simulink model "vertMotorSimMath"  (R2024b)
settings: Solver=FixedStepDiscrete  StartTime=0.0  StopTime=inf  FixedStep=0.002  RelTol=1e-3  EnableMultiTasking=on
undefined symbols (not defined in the file or in its folder): prop, rad, s
libraries: aerolibconvert2 x1
settings Model: ExtModeTrigDuration=10000  Creator=jellu  LastModifiedBy=jellu
settings SolverCC: AlgebraicLoopSolver=TrustRegion  PositivePriorityOrder=on
settings DataIOCC: ReturnWorkspaceOutputs=off
settings OptimizationCC: LifeSpan=inf
settings DebuggingCC: UnconnectedInputMsg=warning  UnconnectedOutputMsg=warning  UnconnectedLineMsg=warning  ArithmeticOperatorsInVariantConditions=warning
settings ModelReferenceCC: EnableRefExpFcnMdlSchedulingChecks=on
settings SFSimCC: SimUseLocalCustomCode=off  CustomCodeUndefinedFunction=UseInterfaceOnly
settings RTWCC: Description=QUARC Win64 Target  SystemTargetFile=quarc_win64.tlc  TemplateMakefile=quarc_default_tmf  RTWUseLocalCustomCode=off  GPUComputeCapability=3.5
settings CodeAppCC: StateflowObjectComments=on
settings STFCustomTargetCC: TargetPreCompLibLocation=C:\PROGRA~3\QUARC\lib\2016a\win64\release  TargetLangStandard=C99 (ISO)  ConcurrentExecutionCompliant=on  GRTInterface=on  SystemTargetFile=quarc_win64.tlc
settings GRTTargetCC: TargetPreCompLibLocation=C:\PROGRA~3\QUARC\lib\2016a\win64\release  ParMdlRefBuildCompliant=off  CompOptLevelCompliant=off  CombineOutputUpdateFcns=off  MatFileLogging=off  CPPClassGenCompliant=off  GRTInterface=on  UseToolchainInfoCompliant=off  ExtMode=on  ExtModeMexFile=quarc_comm
settings ConfigComp: CovMetricSettings=dswe

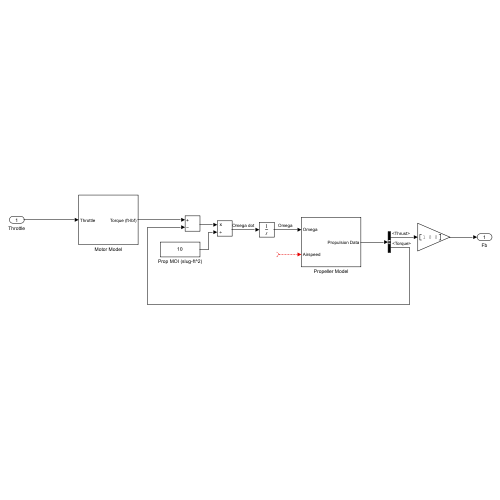
[thumbnail: Simulink's stored preview of the top-level diagram]
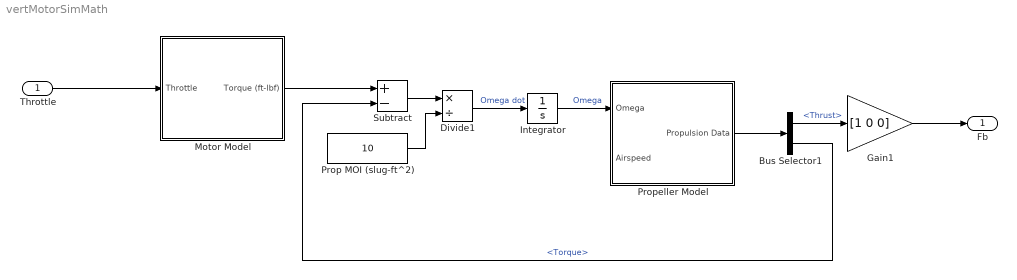
== system vertMotorSimMath ==
  Throttle : Inport
  Bus Selector1 : BusSelector  OutputSignals=Thrust,Torque
  Divide1 : Product  Inputs=*/
  Gain1 : Gain  Gain=[1 0 0]
  Integrator : Integrator  InitialCondition=200
  Motor Model : Subsystem
  Prop MOI (slug-ft^2) : Constant  Value=10
  Propeller Model : Subsystem
  Subtract : Sum  Inputs=+-
  Fb : Outport
  wires:
  Divide1/1 -> Integrator/1  "Omega dot"
  Integrator/1 -> Propeller Model/1(Omega)  "Omega"
  Gain1/1 -> Fb/1
  Motor Model/1(Torque (ft-lbf)) -> Subtract/1
  ? -> Propeller Model/2(Airspeed)
  Bus Selector1/2 -> Subtract/2  "<Torque>"
  Bus Selector1/1 -> Gain1/1  "<Thrust>"
  Prop MOI (slug-ft^2)/1 -> Divide1/2
  Subtract/1 -> Divide1/1
  Propeller Model/1(Propulsion Data) -> Bus Selector1/1
  Throttle/1 -> Motor Model/1(Throttle)

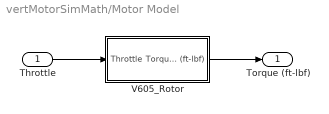
== system vertMotorSimMath/Motor Model ==
  Throttle : Inport
  V605_Rotor : Subsystem
  Torque (ft-lbf) : Outport
  wires:
  V605_Rotor/1(Torque (ft-lbf)) -> Torque (ft-lbf)/1
  Throttle/1 -> V605_Rotor/1(Throttle)

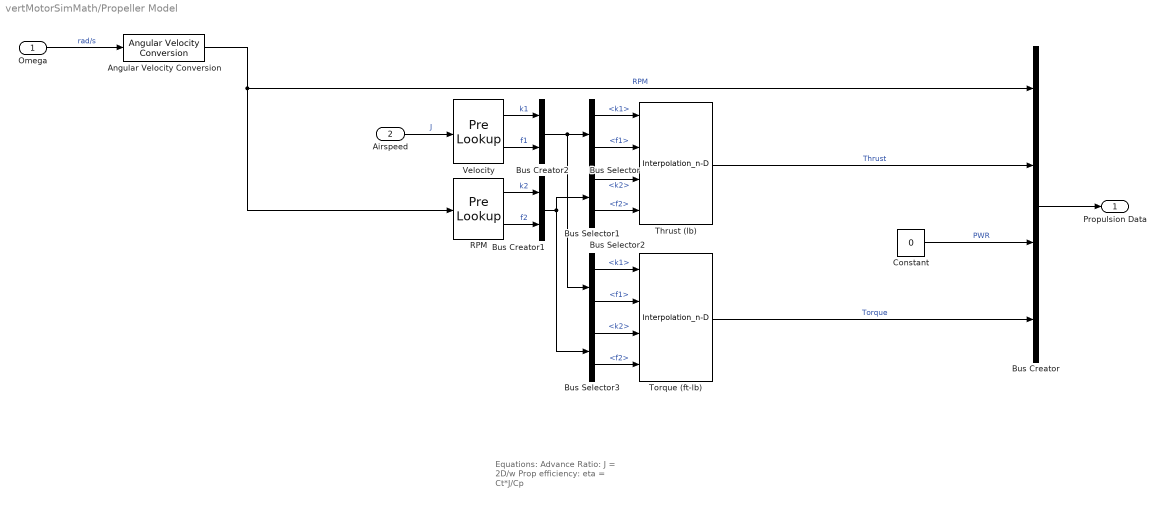
== system vertMotorSimMath/Propeller Model ==
  note: Equations:
      |
      | Advance Ratio: J = 2D/w
      | Prop efficiency: eta = Ct*J/Cp
  Omega : Inport
  Airspeed : Inport  Port=2
  Angular Velocity Conversion : aerolibconvert2/Angular Velocity Conversion  IU=rad/s  OU=rpm
  Bus Creator : BusCreator  Inputs=4
  Bus Creator1 : BusCreator  Inputs=2
  Bus Creator2 : BusCreator  Inputs=2
  Bus Selector : BusSelector  OutputSignals=k1,f1
  Bus Selector1 : BusSelector  OutputSignals=k2,f2
  Bus Selector2 : BusSelector  OutputSignals=k1,f1
  Bus Selector3 : BusSelector  OutputSignals=k2,f2
  Constant : Constant  Value=0
  RPM : PreLookup  BreakpointsData=prop.RPM  ExtrapMethod=Linear
  Thrust (lb) : Interpolation_n-D  Table=prop.Thrust  InternalRulePriority=Speed
  Torque (ft-lb) : Interpolation_n-D  Table=prop.Torque  ExtrapMethod=Clip  InternalRulePriority=Speed
  Velocity : PreLookup  BreakpointsData=prop.vel
  Propulsion Data : Outport
  wires:
  Constant/1 -> Bus Creator/3  "PWR"
  Torque (ft-lb)/1 -> Bus Creator/4  "Torque"
  Angular Velocity Conversion/1 -> RPM/1, Bus Creator/1  "RPM"
  Bus Creator/1 -> Propulsion Data/1
  Omega/1 -> Angular Velocity Conversion/1  "rad/s"
  Airspeed/1 -> Velocity/1  "J"
  Velocity/2 -> Bus Creator2/2  "f1"
  Bus Creator2/1 -> Bus Selector/1, Bus Selector2/1
  Bus Creator1/1 -> Bus Selector1/1, Bus Selector3/1
  Velocity/1 -> Bus Creator2/1  "k1"
  Bus Selector2/2 -> Torque (ft-lb)/2  "<f1>"
  RPM/1 -> Bus Creator1/1  "k2"
  Bus Selector2/1 -> Torque (ft-lb)/1  "<k1>"
  RPM/2 -> Bus Creator1/2  "f2"
  Thrust (lb)/1 -> Bus Creator/2  "Thrust"
  Bus Selector/2 -> Thrust (lb)/2  "<f1>"
  Bus Selector3/2 -> Torque (ft-lb)/4  "<f2>"
  Bus Selector/1 -> Thrust (lb)/1  "<k1>"
  Bus Selector1/2 -> Thrust (lb)/4  "<f2>"
  Bus Selector3/1 -> Torque (ft-lb)/3  "<k2>"
  Bus Selector1/1 -> Thrust (lb)/3  "<k2>"

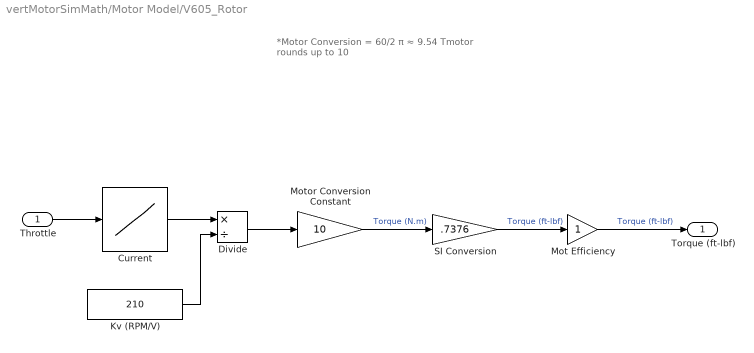
== system vertMotorSimMath/Motor Model/V605_Rotor ==
  note: *Motor Conversion = 60/2 π ≈ 9.54
      | Tmotor rounds up to 10
  Throttle : Inport
  Current : Lookup_n-D  NumberOfTableDimensions=1  BreakpointsForDimension1=[0;2;4;6;8;10;12;14;16;18;20;22;24;26;28;30;32;34;36;38;40;42;44;46;48;50;52;54;56;58;60;62;64;66;68;70;80;90;100]  Table=[0;0.36049999999999999;0.72099999999999997;1.0814999999999999;1.4419999999999999;1.8025;2.1629999999999998;2.5234999999999999;2.8839999999999999;3.2444999999999999;3.605;3.9655;4.3259999999999996;4.6864999999999997;5.0469999999999997;5.4074999999999998;5.7679999999999998;6.1284999999999998;6.4889999999999999;6.8494999999999999;7.21;8.1999999999999993;9.0899999999999999;10.289999999999999;11.56;12.94;14.119999999999999;15.460000000000001;16.760000000000002;18;19.460000000000001;21.059999999999999;22.609999999999999;24.510000000000002;26.190000000000001;28.109999999999999;38.689999999999998;52.159999999999997;68.299999999999997]  InternalRulePriority=Speed  RndMeth=Simplest
  Divide : Product  Inputs=*/
  Kv (RPM/V) : Constant  Value=210
  Mot Efficiency : Gain
  Motor Conversion Constant : Gain  Gain=10
  SI Conversion : Gain  Gain=.7376
  Torque (ft-lbf) : Outport
  wires:
  Divide/1 -> Motor Conversion Constant/1
  Kv (RPM/V)/1 -> Divide/2
  Current/1 -> Divide/1
  SI Conversion/1 -> Mot Efficiency/1  "Torque (ft-lbf)"
  Mot Efficiency/1 -> Torque (ft-lbf)/1  "Torque (ft-lbf)"
  Motor Conversion Constant/1 -> SI Conversion/1  "Torque (N.m)"
  Throttle/1 -> Current/1
